simulink model "REG"  (R2020a)
settings: Solver=VariableStepAuto  StartTime=0.0  StopTime=10.0  RelTol=1e-3
model workspace (MAT data in the model file):
  phi_1_param = Simulink.Parameter
  phi_1_param.Value = [1; 1; 1]
  phi_1_param.DataType = 'auto'
  phi_1_param.Dimensions = [3 1]
  theta_1_param = Simulink.Parameter
  theta_1_param.Value = [1; 1; 1]
  theta_1_param.DataType = 'auto'
  theta_1_param.Dimensions = [3 1]
settings Model: ParameterArgumentNames=phi_1_param,theta_1_param  OrderedModelArguments=off  Creator=andrey  LastModifiedBy=andrey

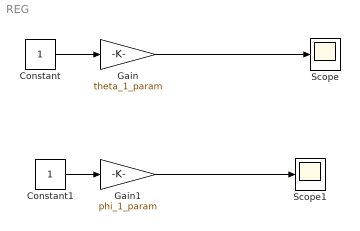
== system REG ==
  Constant : Constant
  Constant1 : Constant
  Gain : Gain  Gain=theta_1_param
  Gain1 : Gain  Gain=phi_1_param
  Scope : Scope
  Scope1 : Scope
  wires:
  Gain/1 -> Scope/1
  Constant/1 -> Gain/1
  Constant1/1 -> Gain1/1
  Gain1/1 -> Scope1/1
